simulink model "Eanom"  (R2018b)
settings: Solver=FixedStepAuto  StartTime=0.0  StopTime=Ts  FixedStep=dt  RelTol=1e-3
values from neighbouring files (symbols this model uses):
  dUT1 = 196.5014E-3    (= 0.1965014)    [AA203_final.m]
  e = sqrt(vec_e(1)^2+vec_e(2)^2+vec_e(3)^2)    [AA203_final.m]
  ep = (mag_v^2)/2-(mu/mag_r)    [AA203_final.m]
  in = in/pi()*180    [AA203_final.m]
  lam_gs = 0    [AA203_final.m]
  M = Mo    [AA203_final.m]
  MJD = 365*y - 679004 + floor(B) + floor(30.6001*(m+1)) + D    [AA203_final.m]
  n = sqrt(mu/a^3)    [AA203_final.m]
  o = o/pi()*180    [AA203_final.m]
  p = mag_h^2/mu    [AA203_final.m]
  phi_gs = 0    [AA203_final.m]
  R_gs_ECEF = zeros(1,3)    [AA203_final.m]
  w = w/pi()*180    [AA203_final.m]
settings Model: Creator=ronik  LastModifiedBy=ronik

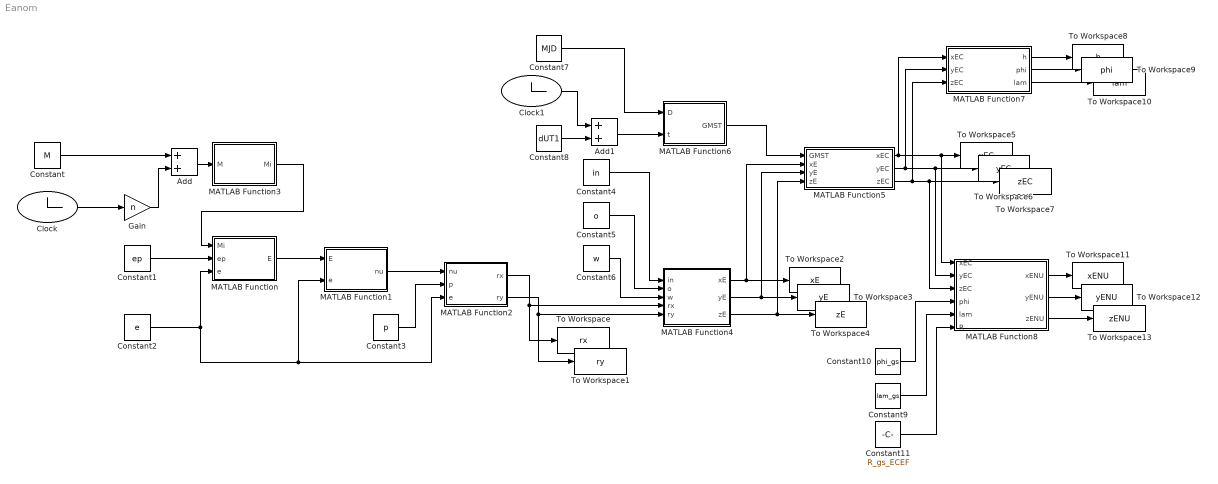
== system Eanom ==
  Add : Sum
  Add1 : Sum
  Clock : Clock
  Clock1 : Clock
  Constant : Constant  Value=M
  Constant1 : Constant  Value=ep
  Constant10 : Constant  Value=phi_gs
  Constant11 : Constant  Value=R_gs_ECEF
  Constant2 : Constant  Value=e
  Constant3 : Constant  Value=p
  Constant4 : Constant  Value=in
  Constant5 : Constant  Value=o
  Constant6 : Constant  Value=w
  Constant7 : Constant  Value=MJD
  Constant8 : Constant  Value=dUT1
  Constant9 : Constant  Value=lam_gs
  Gain : Gain  Gain=n
  MATLAB Function : MATLAB Function  TreatAsAtomicUnit=on
  MATLAB Function1 : MATLAB Function  TreatAsAtomicUnit=on
  MATLAB Function2 : MATLAB Function  TreatAsAtomicUnit=on
  MATLAB Function3 : MATLAB Function  TreatAsAtomicUnit=on
  MATLAB Function4 : MATLAB Function  TreatAsAtomicUnit=on
  MATLAB Function5 : MATLAB Function  TreatAsAtomicUnit=on
  MATLAB Function6 : MATLAB Function  TreatAsAtomicUnit=on
  MATLAB Function7 : MATLAB Function  TreatAsAtomicUnit=on
  MATLAB Function8 : MATLAB Function  TreatAsAtomicUnit=on
  To Workspace : ToWorkspace  VariableName=rx  SampleTime=-1
  To Workspace1 : ToWorkspace  VariableName=ry  SampleTime=-1
  To Workspace10 : ToWorkspace  VariableName=lam  SampleTime=-1
  To Workspace11 : ToWorkspace  VariableName=xENU  SampleTime=-1
  To Workspace12 : ToWorkspace  VariableName=yENU  SampleTime=-1
  To Workspace13 : ToWorkspace  VariableName=zENU  SampleTime=-1
  To Workspace2 : ToWorkspace  VariableName=xE  SampleTime=-1
  To Workspace3 : ToWorkspace  VariableName=yE  SampleTime=-1
  To Workspace4 : ToWorkspace  VariableName=zE  SampleTime=-1
  To Workspace5 : ToWorkspace  VariableName=xEC  SampleTime=-1
  To Workspace6 : ToWorkspace  VariableName=yEC  SampleTime=-1
  To Workspace7 : ToWorkspace  VariableName=zEC  SampleTime=-1
  To Workspace8 : ToWorkspace  VariableName=h  SampleTime=-1
  To Workspace9 : ToWorkspace  VariableName=phi  SampleTime=-1
  wires:
  Clock/1 -> Gain/1
  Constant/1 -> Add/1
  Gain/1 -> Add/2
  Constant1/1 -> MATLAB Function/2(ep)
  MATLAB Function/1(E) -> MATLAB Function1/1(E)
  Constant2/1 -> MATLAB Function1/2(e), MATLAB Function2/3(e), MATLAB Function/3(e)
  MATLAB Function1/1(nu) -> MATLAB Function2/1(nu)
  Constant3/1 -> MATLAB Function2/2(p)
  MATLAB Function2/1(rx) -> To Workspace/1, MATLAB Function4/4(rx)
  MATLAB Function2/2(ry) -> To Workspace1/1, MATLAB Function4/5(ry)
  Add/1 -> MATLAB Function3/1(M)
  MATLAB Function3/1(Mi) -> MATLAB Function/1(Mi)
  Constant4/1 -> MATLAB Function4/1(in)
  Constant5/1 -> MATLAB Function4/2(o)
  Constant6/1 -> MATLAB Function4/3(w)
  MATLAB Function4/1(xE) -> MATLAB Function5/2(xE), To Workspace2/1
  MATLAB Function4/2(yE) -> MATLAB Function5/3(yE), To Workspace3/1
  MATLAB Function4/3(zE) -> MATLAB Function5/4(zE), To Workspace4/1
  MATLAB Function5/1(xEC) -> To Workspace5/1, MATLAB Function8/1(xEC), MATLAB Function7/1(xEC)
  MATLAB Function5/2(yEC) -> MATLAB Function8/2(yEC), To Workspace6/1, MATLAB Function7/2(yEC)
  MATLAB Function5/3(zEC) -> MATLAB Function8/3(zEC), To Workspace7/1, MATLAB Function7/3(zEC)
  MATLAB Function6/1(GMST) -> MATLAB Function5/1(GMST)
  Constant7/1 -> MATLAB Function6/1(D)
  Constant8/1 -> Add1/2
  Add1/1 -> MATLAB Function6/2(t)
  Clock1/1 -> Add1/1
  MATLAB Function7/1(h) -> To Workspace8/1
  MATLAB Function7/2(phi) -> To Workspace9/1
  MATLAB Function7/3(lam) -> To Workspace10/1
  Constant10/1 -> MATLAB Function8/4(phi)
  Constant9/1 -> MATLAB Function8/5(lam)
  MATLAB Function8/1(xENU) -> To Workspace11/1
  MATLAB Function8/2(yENU) -> To Workspace12/1
  MATLAB Function8/3(zENU) -> To Workspace13/1
  Constant11/1 -> MATLAB Function8/6(R)

== matlab function Eanom/MATLAB Function1 ==
  data: E input; nu output; e input
function nu = E2v(E,e)
    nu = acos((cos(E)-e)/(1-e*cos(E)));
    if E > pi()
        nu = 2*pi() - nu;
    end
end

== matlab function Eanom/MATLAB Function ==
  data: Mi input; ep input; E output; e input
function E  = Eanom(Mi,ep,e)
    Ei = Mi;
    Ei1 = Ei-(Ei-e*sin(Ei)-Mi)/(1-e*cos(Ei));
    while (abs(Ei1-Ei) > ep)
        Ei = Ei1;
        Ei1 = Ei-(Ei-e*sin(Ei)-Mi)/(1-e*cos(Ei));
    end
    E = Ei1;
end

== matlab function Eanom/MATLAB Function2 ==
  data: nu input; p input; e input; rx output; ry output
function [rx,ry] = PQW(nu,p,e)
    nu = transpose(nu);
    r = p./(1+e*cos(nu));
    rx = r.*cos(nu);
    ry = r.*sin(nu);
end

== matlab function Eanom/MATLAB Function3 ==
  data: M input; Mi output
function Mi = M2Mi(M)
    f = floor(M/(2*pi()));
    Mi = M-f*2*pi();
end

== matlab function Eanom/MATLAB Function4 ==
  data: in input; xE output; o input; w input; rx input; ry input; yE output; zE output
function [xE,yE,zE] = Per2ECI(in,o,w,rx,ry)
    RP2ECI = rotz(o)*rotx(in)*rotz(w);
    xE = zeros(length(rx));
    yE = zeros(length(rx));
    zE = zeros(length(rx));
    for i = 1:length(rx)
        R = [rx(i) ry(i) 0];
        R = RP2ECI*transpose(R);
        xE(i) = R(1);
        yE(i) = R(2);
        zE(i) = R(3);
    end
end

== matlab function Eanom/MATLAB Function5 ==
  data: GMST input; xEC output; xE input; yE input; zE input; yEC output; zEC output
function [xEC,yEC,zEC] = CRF2TRF(GMST,xE,yE,zE)
    Rot = rotz(-GMST);
    xEC = zeros(length(xE));
    yEC = zeros(length(yE));
    zEC = zeros(length(zE));
    for i = 1:length(xE)
        R = [xE(i) yE(i) zE(i)];
        R = Rot*transpose(R);
        xEC(i) = R(1);
        yEC(i) = R(2);
        zEC(i) = R(3);
    end
end

== matlab function Eanom/MATLAB Function6 ==
  data: D input; GMST output; t input
function GMST = MJD2GMST(D,t)
    J2000 = 51543 + 1.5;
    D = D + t/(3600*24);
    d = D - J2000;
    the = 280.4606 + 360.9856473*d;
    f = floor(the/360);
    GMST = the-f*360;
end

== matlab function Eanom/MATLAB Function7 ==
  data: xEC input; h output; yEC input; zEC input; phi output; lam output
function [h,phi,lam] = ECEF2gd(xEC,yEC,zEC)
    
    lam = zeros(length(xEC));
    phi = zeros(length(xEC));
    h = zeros(length(xEC));
    
    for i = 1:length(xEC)
        R = [xEC(i), yEC(i), zEC(i)];
        rE = 6378.1; % km
        eE = 0.0818;
        lam(i) = atan2(R(2),R(1));
        r = norm(R);

        tol = 10E-10;
        d_phi = 1;
        phi_1 = asin(R(3)/r);
        N_1 = 0;

        while d_phi > tol
            N_1 = rE/sqrt(1-eE^2*sin(phi_1)^2);
            phi_2 = atan2(R(3)+N_1*eE^2*sin(phi_1),sqrt(R(1)^2+R(2)^2));
            d_phi = abs(phi_2-phi_1);
            phi_1 = phi_2;
        end

        phi(i) = phi_1;
        h(i) = sqrt(R(1)^2+R(2)^2)/cos(phi(i))-N_1;
    end
end

== matlab function Eanom/MATLAB Function8 ==
  data: xEC input; xENU output; yEC input; zEC input; phi input; lam input; yENU output; zENU output; R input
function [xENU,yENU,zENU] = ECEF2ENU(xEC,yEC,zEC,phi,lam,R)
    E = [-sin(lam) cos(lam) 0];
    E = transpose(E);
    N = [-sin(phi)*cos(lam) -sin(phi)*sin(lam) cos(phi)];
    N = transpose(N);
    U = [cos(phi)*cos(lam) cos(phi)*sin(lam) sin(phi)];
    U = transpose(U);
    Rot = zeros(3,3);
    xENU = zeros(length(xEC));
    yENU = zeros(length(xEC));
    zENU = zeros(length(xEC));
    Rot(1:3,1) = E;
    Rot(1:3,2) = N;
    Rot(1:3,3) = U;
    for i = 1:length(xEC)
        rEC = [xEC(i); yEC(i); zEC(i)];
        rENU = transpose(Rot)*(rEC-R);
        xENU(i) = rENU(1);
        yENU(i) = rENU(2);
        zENU(i) = rENU(3);
    end
end
